simulink model "kundur_synchronous_machine"  (R2025a)
settings: Solver=VariableStepAuto  StartTime=0.0  StopTime=4  RelTol=1e-3
libraries: spsSynchronousMachinepuStandardLib x1, spsThreePhaseSourceLib x1, sps_lib x1
settings Model: Creator=psernatorre  LastModifiedBy=psernatorre

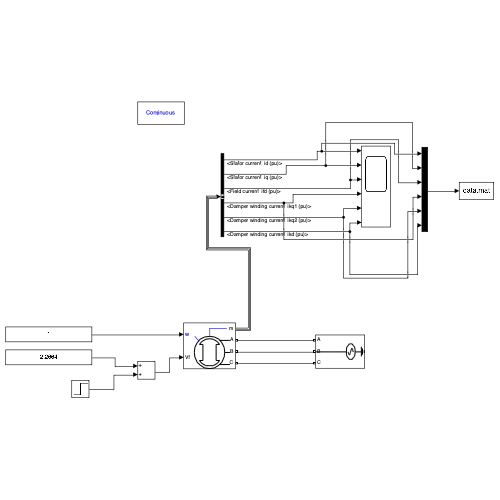
[thumbnail: Simulink's stored preview of the top-level diagram]
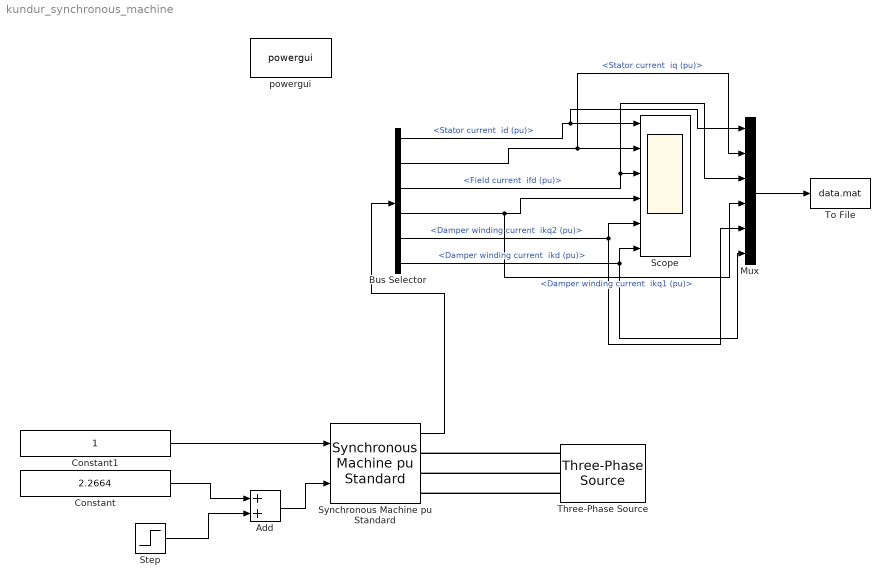
== system kundur_synchronous_machine ==
  Add : Sum
  Bus Selector : BusSelector  OutputSignals="dq0 components.Stator current  id (pu),dq0 components.Stator current  iq (pu),dq0 components.Field current  ifd (pu),dq0 components.Damper winding current  ikq1 (pu),dq0 components.Damper winding current  ikq2 (pu),dq0 components.Damper winding current  ikd (pu)"
  Constant : Constant  Value=2.2664
  Constant1 : Constant
  Mux : Mux  Inputs=6
  Scope : Scope  NumInputPorts=6
      settings: ActiveDisplayYMinimum=0.45162193523490529  ActiveDisplayYMaximum=0.4522256294508113
  Step : Step  After=0.5  SampleTime=0
  Synchronous Machine pu Standard : spsSynchronousMachinepuStandardLib/Synchronous Machine pu Standard  PresetModel=No  MechanicalLoad=Speed w  ShowDetailedParameters=on  RotorType=Round  Units=per unit standard parameters  MeasurementBus=off  NominalParameters=[100e6 480 60]  Reactances1=[ 1.81, 0.30, 0.23, 1.76, 0.65, 0.25, 0.15 ]  Reactances2=[2.24 0.17 0.12 1.02 0.13 0.08]  dAxisTimeConstants=Open-circuit  qAxisTimeConstants=Open-circuit  TimeConstants1="[ 4.4849  0.0681  0.1  ]"  TimeConstants2=[ 8.0, 0.03, 1.0, 0.07 ]  TimeConstants3="[  4.49  0.0681  0.0513  ]"  TimeConstants4=[ 8.0, 0.03, 0.3371, 0.0295 ]  TimeConstants5=[ 1.01, 0.053, 0.1 ]  TimeConstants6=[ 1.3201, 0.023, 1.0, 0.07 ]  TimeConstants7=[0.012 0.003 0.003]  TimeConstants8=[ 1.3201, 0.0231, 0.3371, 0.0295 ]  StatorResistance=0.003  Mechanical=[0.1028 0.02056 2]  PolePairs=2  InitialConditions=[0 -37.6016 1.0198 1.0198 1.0198 -11.3099 -131.31 108.69 2.26642]  SetSaturation=off  Saturation=[0.6404,0.7127,0.8441,0.9214,0.9956,1.082,1.19,1.316,1.457;0.7,0.7698,0.8872,0.9466,0.9969,1.046,1.1,1.151,1.201]  LoadFlowParameters=[1,0,0,0,0]  TsPowergui=0  TsBlock=-1  IterativeModel=Trapezoidal non iterative  IterativeDiscreteModel=Trapezoidal non iterative  BusType=PQ  Pref=100000000  Qref=20000000  Qmin=20000000  Qmax=Inf  PLF=0  QLF=0
  Three-Phase Source : spsThreePhaseSourceLib/Three-Phase Source  InternalConnection=Yg  VoltagePhases=off  Voltage=(480)*1  PhaseAngle=0  Voltage_phases=[25e3 25e3 25e3]/sqrt(3)  PhaseAngles_phases=[0 -120 +120]  Frequency=60  NonIdealSource=off  SpecifyImpedance=off  Resistance=0.0001  Inductance=0  ShortCircuitLevel=100e6  BaseVoltage=480  XRratio=7  BusType=swing  Pref=10000  Qref=0  Prefabc=[10e3, 10e3, 10e3]  Qrefabc=[0, 0, 0]  Qmin=-Inf  Qmax=Inf
  To File : ToFile  Filename=data.mat  SaveFormat=Timeseries
  powergui : sps_lib/powergui  Priority=1  SimulationMode=Continuous  SampleTime=50e-6  frequency=60  Iterations=50  frequencyindice=60  Pbase=100e6  ErrMax=1e-4  UnitsV=kV  UnitsW=MW  buscounter=0  FunctionMessages=off  echomessages=off  EnableUseOfTLC=off  CurrentSourceSwitches=off  DisableSnubberDevices=off  DisableRonSwitches=off  DisableVfSwitches=off  DisplayEquations=off  AutomaticDiscreteSolvers=off  SolverType=Tustin/Backward Euler (TBE)  Interpol=off  ExternalGateDelay=off  methode=off  Ts=100  x0status=blocks  SPID=on  SwTol=0  HookPort=off  NonlinearTolerance=1e-4  nMaxIteration=100  ContinueOnMaxIteration=off  RestoreLinks=warning  ResistiveCurrentMeasurement=off  Frange=[0:2:500]  Ylog=off  Xlog=on  ShowGrid=off  save=off  variable=ZData  structure=0  ZoomFFT=off  StartTime=0.0  cycles=1  DisplayStyle=1  fundamental=60  FreqAxis=off  MaxFrequency=1000  frequencyindicesteady=1  RmsSteady=1  display=off
  wires:
  Constant1/1 -> Synchronous Machine pu Standard/1
  Synchronous Machine pu Standard/1 -> Bus Selector/1
  Bus Selector/3 -> Mux/3, Scope/3  "<Field current  ifd (pu)>"
  Bus Selector/6 -> Mux/6, Scope/6  "<Damper winding current  ikd (pu)>"
  Bus Selector/4 -> Mux/4, Scope/4  "<Damper winding current  ikq1 (pu)>"
  Bus Selector/5 -> Mux/5, Scope/5  "<Damper winding current  ikq2 (pu)>"
  Mux/1 -> To File/1
  Constant/1 -> Add/1
  Step/1 -> Add/2
  Add/1 -> Synchronous Machine pu Standard/2
  Bus Selector/2 -> Mux/2, Scope/2  "<Stator current  iq (pu)>"
  Bus Selector/1 -> Mux/1, Scope/1  "<Stator current  id (pu)>"
  connections:
  Three-Phase Source/RConn2 -- Synchronous Machine pu Standard/RConn2
  Three-Phase Source/RConn1 -- Synchronous Machine pu Standard/RConn1
  Three-Phase Source/RConn3 -- Synchronous Machine pu Standard/RConn3
